simulink model "ProjectileMotion_SIM"  (R2012b)
settings: Solver=ode3  StartTime=0.0  StopTime=10.0  FixedStep=0.01  RelTol=1e-3
values from neighbouring files (symbols this model uses):
  k = k_values(m)    [ProjectileMotion.m]
  r0x = r0(1, 1)    [ProjectileMotion.m]
  r0y = r0(2, 1)    [ProjectileMotion.m]
  v0x = v0(1, 1)    [ProjectileMotion.m]
  v0y = v0(2, 1)    [ProjectileMotion.m]
settings Model: Creator=aluno  LastModifiedBy=aluno

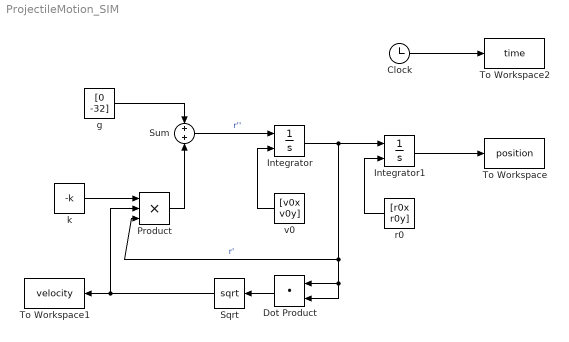
== system ProjectileMotion_SIM ==
  Clock : Clock
  Dot Product : DotProduct  InputSameDT=on  OutDataTypeStr=Inherit: Inherit via internal rule
  Integrator : Integrator  InitialConditionSource=external
  Integrator1 : Integrator  InitialConditionSource=external
  Product : Product  Inputs=3  RndMeth=Zero
  Sqrt : Sqrt  SaturateOnIntegerOverflow=on
  Sum : Sum
  To Workspace : ToWorkspace  VariableName=position  SampleTime=-1
  To Workspace1 : ToWorkspace  VariableName=velocity  SampleTime=-1
  To Workspace2 : ToWorkspace  VariableName=time  SampleTime=-1
  g : Constant  Value=[0 -32]
  k : Constant  Value=-k
  r0 : Constant  Value=[r0x r0y]
  v0 : Constant  Value=[v0x v0y]
  wires:
  Integrator1/1 -> To Workspace/1
  Sum/1 -> Integrator/1  "r''"
  g/1 -> Sum/1
  Product/1 -> Sum/2
  k/1 -> Product/1
  v0/1 -> Integrator/2
  r0/1 -> Integrator1/2
  Integrator/1 -> Dot Product/2, Dot Product/1, Product/3, Integrator1/1  "r'"
  Dot Product/1 -> Sqrt/1
  Sqrt/1 -> To Workspace1/1, Product/2
  Clock/1 -> To Workspace2/1
